simulink model "GMCLIB_ParkInv_BAM_F16"  (Simulink 8.3)
settings: Solver=ode45  StartTime=0.0  StopTime=10.0  RelTol=1e-3
settings Model: Creator=RE004C  LastModifiedBy=B17364
settings OptimizationCC: ExpressionDepthLimit=2147483647
settings DebuggingCC: FcnCallInpInsideContextMsg=UseLocalSettings  StrictBusMsg=Warning
settings HardwareCC: ProdLargestAtomicInteger=Long  ProdLargestAtomicFloat=Double  ProdIntDivRoundTo=Zero  ProdEndianess=BigEndian  ProdHWDeviceType=Freescale->32-bit PowerPC

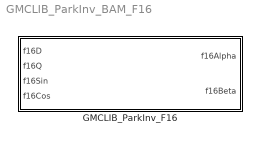
== system GMCLIB_ParkInv_BAM_F16 ==
  GMCLIB_ParkInv_F16 : Subsystem  mask(GMCLIB_ParkInv_F16){}
      mask help: Bit accurate model of Inverse Park transformation 2ph rotational -> 2ph stationary.
      mask init:
      | pos = get_param(gcb, 'Position');width = pos(3) - pos(1); height = pos(4) - pos(2);tX=width/2;tY=height*0.9;
      mask Display: color('black');port_label('input',1,'f16D');port_label('input',2,'f16Q');port_label('input',3,'f16Sin');port_label('input',4,'f16Cos');port_label('output',1,'f16Alpha');port_label('output',2,'f16Beta');color('black');disp('GMCLIB_ParkInv_F16');color('blue');text(tX,tY, 'BAM', 'horizontalAlignment', 'center');

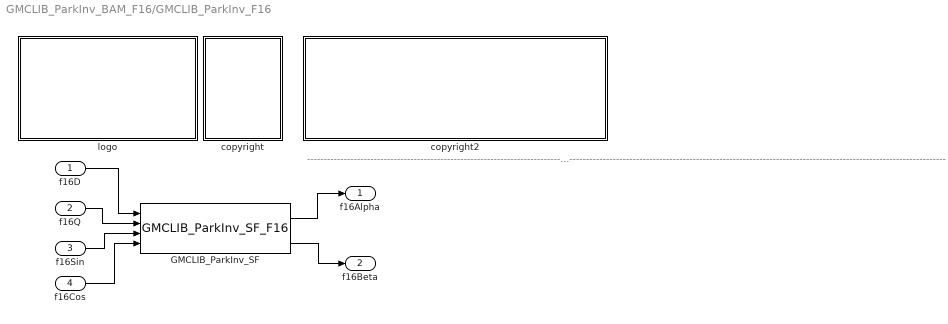
== system GMCLIB_ParkInv_BAM_F16/GMCLIB_ParkInv_F16 ==
  note: ---------------------------------------------------------------------------------------------------------------------------------------------------------------------------------------------------
  f16D : Inport
  f16Q : Inport  Port=2
  f16Sin : Inport  Port=3
  f16Cos : Inport  Port=4
  GMCLIB_ParkInv_SF : S-Function  FunctionName=GMCLIB_ParkInv_SF_F16  EnableBusSupport=off
  copyright : Subsystem
      mask Display:
      | text(10,90,'FILE:');text(10,75,'DESRIPTION:')
      | text(10,60,'COPYRIGHT:')
      | text(10,45,'VERSION:')
      | text(10,30,'DATE:')
  copyright2 : Subsystem
      mask Display:
      | text(10,90,'GMCLIB_ParkInv_BAM_F16.mdl');text(10,75,'Inverse Park transformation.');text(10,60,'Freescale')
      | text(10,45,'0.1');text(10,30,'19-Sep-2011');
  logo : Subsystem
      mask Display: image(imread('logo.jpg'))
  f16Alpha : Outport
  f16Beta : Outport  Port=2
  wires:
  f16D/1 -> GMCLIB_ParkInv_SF/1
  f16Q/1 -> GMCLIB_ParkInv_SF/2
  f16Sin/1 -> GMCLIB_ParkInv_SF/3
  f16Cos/1 -> GMCLIB_ParkInv_SF/4
  GMCLIB_ParkInv_SF/1 -> f16Alpha/1
  GMCLIB_ParkInv_SF/2 -> f16Beta/1

== system GMCLIB_ParkInv_BAM_F16/GMCLIB_ParkInv_F16/copyright ==

== system GMCLIB_ParkInv_BAM_F16/GMCLIB_ParkInv_F16/copyright2 ==

== system GMCLIB_ParkInv_BAM_F16/GMCLIB_ParkInv_F16/logo ==
